simulink model "et_robocon_princess_pi_zack"  (R2013b)
settings: Solver=FixedStepDiscrete  SolverMode=SingleTasking  StartTime=0.0  StopTime=inf  FixedStep=balancer_ts  RelTol=1e-3
undefined symbols (not defined in the file): a_d, a_r, balancerStates_Bus0, Batt, battery_gain, battery_offset, cmd_max, current_mode_status, current_task_operation_status, DiscIntNeverNeededParam, exec_period, Init_Bus0, K, k_f, k_i, k_phidot, k_thetadot, lightCalib, R, see_saw_princess, STATE, TRACK_MODE_LIST, ts2, W
libraries: legonxtlib x29, simulink x19, simulink_extras x4
(part 4 of 4)

== system et_robocon_princess_pi_zack/Main Controller/normal_operation_modes.line_tracking_before_seesaw/line_tracking_mode.Track.lineTracker/SwitchForFreeSteering/tmpController/Derivative ==
  In : Inport
  Constant2 : Constant  Value=Ts_  OutDataTypeStr=single  SampleTime=-1
  Difference : simulink/Discrete/Difference  ICPrevInput=0.0  InputProcessing=Inherited  OutMin=[]  OutMax=[]  OutDataTypeStr=single  OutputDataTypeScalingMode=single  OutDataType=sfix(16)  OutScaling=2^-10  RndMeth=Nearest  DoSatur=off
  Divide4 : Product  Inputs=*/  OutDataTypeStr=single  RndMeth=Nearest
  Out : Outport
  wires:
  Constant2/1 -> Divide4/2
  Divide4/1 -> Difference/1
  In/1 -> Divide4/1
  Difference/1 -> Out/1

== system et_robocon_princess_pi_zack/Main Controller/normal_operation_modes.line_tracking_before_seesaw/line_tracking_mode.Track.lineTracker/SwitchForFreeSteering/tmpController/Fillter ==
  In : Inport
  In1 : Inport  Port=2
  Add : Sum  RndMeth=Nearest
  Add2 : Sum  Inputs=+-  OutDataTypeStr=single  RndMeth=Nearest
  Constant : Constant  Value=single(1-(0.0001/(0.1*Ts_)))  OutDataTypeStr=single  SampleTime=-1
  Constant1 : Constant  Value=single(0.0001/(0.1*Ts_))  OutDataTypeStr=single  SampleTime=-1
  Constant2 : Constant  Value=(0.1*Ts_)  OutDataTypeStr=single  SampleTime=-1
  Constant3 : Constant  OutDataTypeStr=single  SampleTime=-1
  Constant4 : Constant  Value=0.00001  OutDataTypeStr=single  SampleTime=-1
  Constant6 : Constant  Value=(0.1*Ts_)  OutDataTypeStr=single  SampleTime=-1
  Divide : Product  Inputs=*/
  Divide1 : Product  Inputs=*/
  Manual Switch1 : ManualSwitch  CurrentSetting=0
  Manual Switch3 : ManualSwitch  CurrentSetting=0
  Product : Product  OutDataTypeStr=single  RndMeth=Nearest
  Product1 : Product  OutDataTypeStr=single  RndMeth=Nearest
  Product3 : Product  OutDataTypeStr=single  RndMeth=Nearest
  Unit Delay : UnitDelay  SampleTime=-1
  Unit Delay1 : UnitDelay  SampleTime=-1
  Out : Outport
  wires:
  In/1 -> Unit Delay1/1
  Unit Delay1/1 -> Product1/1
  Product1/1 -> Add/1
  Unit Delay/1 -> Product/2
  Add/1 -> Out/1, Unit Delay/1
  Product/1 -> Add/2
  Constant6/1 -> Divide/2
  Constant2/1 -> Divide1/2
  Divide1/1 -> Add2/2
  In1/1 -> Product3/1
  Product3/1 -> Divide1/1, Divide/1
  Constant4/1 -> Product3/2
  Constant3/1 -> Add2/1
  Manual Switch1/1 -> Product1/2
  Constant1/1 -> Manual Switch1/1
  Divide/1 -> Manual Switch1/2
  Manual Switch3/1 -> Product/1
  Constant/1 -> Manual Switch3/1
  Add2/1 -> Manual Switch3/2

== system et_robocon_princess_pi_zack/Main Controller/normal_operation_modes.line_tracking_before_seesaw/line_tracking_mode.Track.lineTracker/SwitchForFreeSteering/tmpController/I_over_guard ==
  In1 : Inport
  Compare To Constant1 : simulink/Logic and Bit Operations/Compare To Constant  relop===  const=1  OutDataTypeStr=uint8
  Constant2 : Constant  Value=0  OutDataTypeStr=uint8  SampleTime=-1
  Constant4 : Constant  Value=0  OutDataTypeStr=uint8  SampleTime=-1
  Memory1 : Memory  X0=1  InheritSampleTime=on
  Switch : Switch  Threshold=1
  Out1 : Outport
  wires:
  Memory1/1 -> Compare To Constant1/1
  Constant2/1 -> Memory1/1
  Constant4/1 -> Switch/1
  Compare To Constant1/1 -> Switch/2
  Switch/1 -> Out1/1
  In1/1 -> Switch/3

== system et_robocon_princess_pi_zack/Main Controller/normal_operation_modes.line_tracking_before_seesaw/line_tracking_mode.Track.lineTracker/SwitchForFreeSteering/tmpController/Integrator ==
  In : Inport
  Constant2 : Constant  Value=Ts_  OutDataTypeStr=single  SampleTime=-1
  Integrator : DiscreteTransferFcn  Denominator=[1 -1]  RndMeth=Nearest
  Product1 : Product  OutDataTypeStr=single  RndMeth=Nearest
  Out : Outport
  wires:
  Constant2/1 -> Product1/2
  Product1/1 -> Integrator/1
  In/1 -> Product1/1
  Integrator/1 -> Out/1

== system et_robocon_princess_pi_zack/Main Controller/normal_operation_modes.line_tracking_before_seesaw/line_tracking_mode.balanceControl/ForSimulation/Cal_PWM/Cal_vol_max ==
  battery : Inport
  Constant : Constant  Value=battery_offset  OutDataTypeStr=single  SampleTime=-1
      settings: AttributesFormatString=DataType = %<OutDataTypeStr>
  Gain3 : Gain  Gain=battery_gain  OutDataTypeStr=Inherit: Same as input  ParamDataTypeStr=Inherit: Same as input
  Sum2 : Sum  Inputs=|+-  OutDataTypeStr=Inherit: Same as first input
  vol_max : Outport
  wires:
  Constant/1 -> Sum2/2
  Sum2/1 -> vol_max/1  "base_pwm"
  Gain3/1 -> Sum2/1
  battery/1 -> Gain3/1

== system et_robocon_princess_pi_zack/Main Controller/normal_operation_modes.line_tracking_before_seesaw/line_tracking_mode.balanceControl/ForSimulation/Cal_Reference/DiscreteIntegrator ==
  in : Inport
  Gain : Gain  Gain=exec_period  OutDataTypeStr=Inherit: Same as input  ParamDataTypeStr=Inherit: Same as input
  Sum : Sum  Inputs=|++  OutDataTypeStr=Inherit: Same as first input
  Unit Delay : UnitDelay  SampleTime=-1  StateName=ud_theta_ref  StateMustResolveToSignalObject=on
      settings: AttributesFormatString=Signal name = ud_theta_ref
  out : Outport
  wires:
  Unit Delay/1 -> Sum/2, out/1
  Gain/1 -> Sum/1
  Sum/1 -> Unit Delay/1
  in/1 -> Gain/1

== system et_robocon_princess_pi_zack/Main Controller/normal_operation_modes.line_tracking_before_seesaw/line_tracking_mode.balanceControl/ForSimulation/Cal_Reference/LowPathFilter ==
  note: Low Path Filter Function
      |               1-a_r
      |          ----------------
      |          1-a_r*z^(-1)
  in : Inport
  Constant : Constant  OutDataTypeStr=single
      settings: AttributesFormatString=DataType = %<OutDataTypeStr>
  Constant1 : Constant  Value=a_r  OutDataTypeStr=single
      settings: AttributesFormatString=DataType = %<OutDataTypeStr>
  Gain2 : Gain  Gain=a_r  OutDataTypeStr=Inherit: Same as input  ParamDataTypeStr=Inherit: Same as input
  Product : Product  RndMeth=Zero
  Sum : Sum  Inputs=|++  OutDataTypeStr=Inherit: Same as first input
  Sum1 : Sum  Inputs=|+-
  Unit Delay : UnitDelay  SampleTime=-1  StateName=ud_thetadot_cmd_lpf  StateMustResolveToSignalObject=on
      settings: AttributesFormatString=Signal name = ud_thetadot_cmd_lpf
  out : Outport
  wires:
  Sum/1 -> Unit Delay/1, out/1
  Unit Delay/1 -> Gain2/1
  Gain2/1 -> Sum/2
  Product/1 -> Sum/1
  in/1 -> Product/1
  Constant/1 -> Sum1/1
  Sum1/1 -> Product/2
  Constant1/1 -> Sum1/2

== system et_robocon_princess_pi_zack/Main Controller/normal_operation_modes.line_tracking_before_seesaw/line_tracking_mode.balanceControl/ForSimulation/Cal_x1/DiscreteDerivative ==
  in : Inport
  in1 : Inport  Port=2
  Constant : Constant  Value=exec_period  OutDataTypeStr=single
  Product : Product  Inputs=*/  RndMeth=Simplest
  Sum : Sum  Inputs=|+-  OutDataTypeStr=Inherit: Same as first input
  out : Outport
  wires:
  Sum/1 -> Product/1
  in1/1 -> Sum/2
  in/1 -> Sum/1
  Product/1 -> out/1
  Constant/1 -> Product/2

== system et_robocon_princess_pi_zack/Main Controller/normal_operation_modes.line_tracking_before_seesaw/line_tracking_mode.balanceControl/ForSimulation/Cal_x1/DiscreteIntegrator ==
  in : Inport
  Gain : Gain  Gain=exec_period  OutDataTypeStr=Inherit: Same as input  ParamDataTypeStr=Inherit: Same as input
  Sum : Sum  Inputs=|++  OutDataTypeStr=Inherit: Same as first input
  Unit Delay : UnitDelay  SampleTime=-1
      settings: AttributesFormatString=Signal name = ud_psi
  out : Outport
  wires:
  Unit Delay/1 -> Sum/2, out/1
  Gain/1 -> Sum/1
  Sum/1 -> Unit Delay/1
  in/1 -> Gain/1

== system et_robocon_princess_pi_zack/Main Controller/normal_operation_modes.line_tracking_before_seesaw/line_tracking_mode.balanceControl/ForSimulation/Cal_x1/LowPathFilter ==
  note: Low Path Filter Function
      |               1-a_d
      |          ----------------
      |          1-a_d*z^(-1)
  in : Inport
  Constant : Constant  OutDataTypeStr=single
      settings: AttributesFormatString=DataType = %<OutDataTypeStr>
  Constant1 : Constant  Value=a_d  OutDataTypeStr=single
      settings: AttributesFormatString=DataType = %<OutDataTypeStr>
  Gain2 : Gain  Gain=a_d  OutDataTypeStr=Inherit: Same as input  ParamDataTypeStr=Inherit: Same as input
  Product : Product  RndMeth=Zero
  Sum : Sum  Inputs=|++  OutDataTypeStr=Inherit: Same as first input
  Sum1 : Sum  Inputs=|+-
  Unit Delay : UnitDelay  SampleTime=-1  StateName=ud_theta_lpf  StateMustResolveToSignalObject=on
      settings: AttributesFormatString=Signal name = ud_thta_lpf
  out : Outport
  out1 : Outport  Port=2
  wires:
  Constant1/1 -> Sum1/2
  Sum1/1 -> Product/2
  Constant/1 -> Sum1/1
  in/1 -> Product/1
  Product/1 -> Sum/1
  Gain2/1 -> Sum/2
  Unit Delay/1 -> Gain2/1, out1/1
  Sum/1 -> out/1, Unit Delay/1  "theta_lpf"

== stateflow chart et_robocon_princess_pi_zack/State Estimation/Gyro Processing/Reset Subsystem ==
  state CheckForReset
    bind: doProcess;
    entry: doProcess;
    during: doProcess;
  (default) -> CheckForReset
  CheckForReset -> CheckForReset : [init_flag == 1]
  data: init_flag input
  events: doProcess output FUNCTION_CALL_EVENT

== stateflow chart et_robocon_princess_pi_zack/State Estimation/StateEstimation/Reset Subsystem ==
  state CheckForReset
    bind: doProcess;
    entry: doProcess;
    during: doProcess;
  (default) -> CheckForReset
  CheckForReset -> CheckForReset : [init_flag == 1]
  data: init_flag input
  events: doProcess output FUNCTION_CALL_EVENT

== stateflow chart et_robocon_princess_pi_zack/Main Controller/normal_operation_modes.see_saw_princess ==
  state see_saw_mode
    entry:
    desired_tail = single(1.6);
    during:
    normalizedLight = processLight(sensors.light,lightCalib);
    PWM.tail = tail_controller(sensors.theta_T, desired_tail);
    DispVar(normalizedLight);
    state light = processLight(rawLight,lightCalib) [function]
    state cmd = phiController(phi,desiredPhi,battery) [function]
    state Balancing
      state SeesawLogic [parallel]
        settings: executionOrder=1
        state StationnaryBalance
          entry:
          debugFlag = uint16(603);
          desired_tail = single(0.5);
          initFlags.theta = single(0);
          initFlags.gyroReset = single(0);
          desired_states = balancerStates_Bus0;
          phi0 = states.phi;
          desired_phi = phi0;
          during:
          %turningPWM = phiController(states.phi,desired_phi,sensors.battery);
          exit:
          turningPWM = single(0);
        state Seesaw
          entry:
          phi0 = states.phi;
          desired_phi = phi0;
          during:
          exit:
          turningPWM = single(0);
          note: % For now I store theta_ref when we receive the bluetooth signal.
              | Eventually one state needs to be added to sear for the ramp
              | and we should store the ref when the ramp is detected.
          state JumpOnIt
            entry:
            debugFlag = uint16(606);
            theta_ref = states.balancerStates.theta;
            des_vel = single(0.16);
            du:
            turningPWM = phiController(states.phi,desired_phi, sensors.battery);
          state ForPhi
            state GoingUP
              en:
              debugFlag = uint16(607);
              des_vel = single(0.1);
              du:
              turningPWM = phiController(states.phi,desired_phi, sensors.battery)+...
              single(3)*lineTracker(single(0.15), normalizedLight, single(1), sensors.battery);
              ex:
              des_vel = single(0);
            state WaitForMario
              en:
              debugFlag = uint16(608);
              des_vel = single(0);
              BT_status_out = single(102);
              du:
              turningPWM =phiController(states.phi,desired_phi, sensors.battery)
            state MoveForward
              en:
              debugFlag = uint16(609);
              des_vel = single(0.005);
              du:
              turningPWM = phiController(states.phi,desired_phi, sensors.battery)+...
              single(3)*lineTracker(single(0.3), normalizedLight, single(1), sensors.battery);
              ex:
              %des_vel = single(0.01);
              state Vel1
                du: des_vel = des_vel + single(0.00024);
              state Vel
                entry:
                des_vel = single(0.06)
                BT_status_out = single(103);
              (default) -> Vel1
              Vel1 -> Vel : [des_vel >= single(0.06)]
            state WaitForMario2
              en:
              debugFlag = uint16(610);
              BT_status_out = single(103);
              du:
              turningPWM =phiController(states.phi,desired_phi, sensors.battery);
            GoingUP -> WaitForMario : [states.balancerStates.theta >= theta_ref + single(5)]
            WaitForMario -> MoveForward : [sensors.BT_status_in == single(3)]
          state GetOff
            entry:
            debugFlag = uint16(611);
            des_vel = single(0);
            during:
            %turningPWM = single(1.1)*lineTracker(single(0.3), normalizedLight, single(1), sensors.battery)+single(1)*phiController(states.phi,desired_phi,sensors.battery);
            turningPWM = phiController(states.phi,desired_phi, sensors.battery);
            exit: des_vel = single(0.04);
          state Stop
            entry:
            debugFlag = uint16(612);
            BT_status_out = single(104);
            du:
            turningPWM = lineTracker(single(0), normalizedLight, single(1), sensors.battery);
            des_vel = des_vel + single(0.0003)
          state Stop1
            entry:
            debugFlag = uint16(613);
            du: turningPWM = lineTracker(single(0), normalizedLight, single(1), sensors.battery)
          (default) -> JumpOnIt
          JumpOnIt -> GoingUP : [states.balancerStates.theta >= theta_ref+single(1.8)]
          MoveForward -> GetOff : [sensors.BT_status_in == single(4)]
          GetOff -> GetOff : [states.balancerStates.theta >= theta_ref + single(30)]
          Stop -> Stop1 : [des_vel >= single(0.08)]
        state RaceDone
          entry: debugFlag = uint16(599);
          current_mode_status = OperationModeStatusEnum.SUCCESSFULLY_COMPLETED;
        (default) -> StationnaryBalance
        StationnaryBalance -> Seesaw
      state After [parallel]
        during:
        forwardPWM = balance_ctrl(states.balancerStates, des_vel ,sensors.battery)
        PWM.left = forwardPWM + turningPWM;
        PWM.right = forwardPWM - turningPWM;
        settings: executionOrder=2
    state cmd = lineTracker(desiredLight,light,trackingPower,battery) [function]
    state Speak [function]
    state cmd = tail_controller(current,desired) [function]
    state cmd = balance_ctrl(balancerStates,desired_velocity,battery) [function]
    state DispVar(Var) [function]
    (default) -> Balancing
  data: rawLight function_input single size=1; lightCalib function_input Bus: Light_Bus size=1; light function_output; cmd function_output; phi function_input single size=1; desiredPhi function_input single size=1; battery function_input double size=1; cmd function_output single size=1; desiredLight function_input single size=1; light function_input single size=1; trackingPower function_input single size=1; battery function_input double size=1; current function_input single size=1; desired function_input single size=1; cmd function_output single size=1; balancerStates function_input Bus: Balancer_States_Bus size=1; desired_velocity function_input single size=1; battery function_input double size=1; cmd function_output single size=1; Var function_input single size=1; states input Bus: States_Bus size=1; sensors input Bus: Sensors_Bus size=1; PWM output Bus: PWM_bus size=1; initFlags output Bus: Init_Bus size=1; debugFlag output uint16 size=1; desired_states local Bus: Balancer_States_Bus size=1; desired_tail local single size=1; current_mode_status data_store_memory; balancerStates_Bus0 parameter Bus: Balancer_States_Bus size=1; lightCalib data_store_memory; normalizedLight local single size=1; des_vel local single size=1; theta_ref local single size=1; forwardPWM local single size=1; turningPWM local single size=1; BT_status_out output single size=1; phi0 local single size=1; desired_phi local single size=1

== stateflow chart et_robocon_princess_pi_zack/Main Controller ==
  state restore
  state emergency_stop
    entry:
    debugFlag = uint16(9999);
  state normal_operation_modes
    state gyro_calibration_mode
    state light_calibration_up
    state line_tracking_before_seesaw
    state see_saw_princess
    state line_tracking_after_seesaw
    state WeShouldNotBeHere
    (default) -> (junction 12) : {
        | current_mode_status = OperationModeStatusEnum.IN_PROGRESS;
        | }
    (junction 12) -> gyro_calibration_mode [order 1] : [  current_mode == OperationModeEnum.GYRO_CALIBRATION ]
    (junction 12) -> (junction 13) [order 2]
    (junction 13) -> ? [order 1] : [ current_mode == OperationModeEnum.LIGHT_CALIBRATION_ON_TAIL ]
    (junction 13) -> (junction 144) [order 1]
    (junction 144) -> light_calibration_up [order 1] : [ current_mode == OperationModeEnum.LIGHT_CALIBRATION_UP ]
    (junction 144) -> (junction 14) [order 2]
    (junction 14) -> line_tracking_before_seesaw [order 2] : [ current_mode == OperationModeEnum.LINE_TRACKING ]
    (junction 14) -> (junction 15) [order 1]
    (junction 15) -> see_saw_princess [order 1] : [ current_mode == OperationModeEnum.SEE_SAW_PRINCESS ]
    (junction 15) -> (junction 17) [order 2]
    (junction 17) -> ? [order 1] : [  current_mode == OperationModeEnum.LIMBO ]
    (junction 17) -> (junction 19) [order 1]
    (junction 19) -> ? [order 1] : [ current_mode == OperationModeEnum.LIGHT_CALIBRATION_LIMBO ]
    (junction 19) -> (junction 140) [order 1]
    (junction 140) -> line_tracking_after_seesaw [order 1] : [ current_mode == OperationModeEnum.LINE_TRACKING_ON_MAP ]
    (junction 140) -> (junction 154) [order 2]
    (junction 154) -> ? [order 1] : [ current_mode == OperationModeEnum.YOSHI ]
    (junction 154) -> (junction 99) [order 1]
    (junction 99) -> WeShouldNotBeHere
  (default) -> (junction 38) : {initFlags = Init_Bus0;BT_status_out = single(0)}
  (junction 37) -> (junction 38)
  (junction 43) -> (junction 37)
  (junction 38) -> (junction 39) : { current_mode_index = uint8( 0 ); }
  (junction 40) -> (junction 39)
  restore -> (junction 40) : [ false == touch ]
  (junction 39) -> (junction 41) : {
      | current_mode_status = OperationModeStatusEnum.NOT_STARTED;
      | }
  normal_operation_modes -> (junction 40) [order 2] : [ current_mode_status == OperationModeStatusEnum.SUCCESSFULLY_COMPLETED ]
  (junction 42) -> (junction 41)
  (junction 41) -> (junction 44) : { current_mode_index = current_mode_index + uint8( 1 ); }
  (junction 47) -> (junction 42)
  emergency_stop -> restore : [ true == touch ]
  (junction 44) -> (junction 43) [order 1] : [ numel( TRACK_MODE_LIST ) < current_mode_index ]
      | % If the "current_mode_index" has exceeded the number
      | % of elements in the list, it should "wrap" back to the start.
  (junction 44) -> (junction 45) [order 2]
  (junction 45) -> (junction 46) : {
      | current_mode = TRACK_MODE_LIST( current_mode_index );
      | }
  (junction 46) -> (junction 47) [order 1] : [  current_mode == OperationModeEnum.SKIP ]
  (junction 46) -> normal_operation_modes [order 2]
  normal_operation_modes -> emergency_stop [order 1] : [ true == fall_detection_input ]
      | {current_mode_status = OperationModeStatusEnum.ABORTED;}
  data: rawSensors input Bus: Sensors_Bus size=1; PWM output Bus: PWM_bus size=1; TRACK_MODE_LIST parameter Enum: OperationModeEnum; current_mode_index local uint8; current_mode data_store_memory; states input Bus: States_Bus size=1; fall_detection_input input boolean size=1; current_mode_status data_store_memory; sensors input Bus: Sensors_Bus size=1; lightCalib data_store_memory; debugFlag output uint16 size=1; BT_status_out output single size=1; touch input single size=1; initFlags output Bus: Init_Bus size=1; Init_Bus0 parameter Bus: Init_Bus size=1; balancerStates_Bus0 parameter Bus: Balancer_States_Bus size=1

== stateflow chart et_robocon_princess_pi_zack/Main Controller/normal_operation_modes.line_tracking_after_seesaw ==
  state line_tracking_mode
    entry:
    desired_tail = single(0); %radian
    entry, during:
    PWM.tail = tail_controller(sensors.theta_T,desired_tail);
    exit:
    PWM.tail = single(0);
    state ResetStates
      entry:
      initFlags.theta = single(1);
      initFlags.gyroReset = single(1);
    state ResetDone
      entry:
      initFlags.theta = single(0);
      initFlags.gyroReset = single(0);
    state Track
      entry:
      debugFlag = uint16(401);
      bias = single(0);
      FlagSteering = single(0);
      minLight = single(-125);
      maxLight = single(-10);
      lineSide = single(1);
      enablePhiTracking = single(0);
      state preProcess [parallel]
        during:
        on every(3, tick):
        [normalizedLight, filteredLight] = processLight(sensors.light, bias, minLight,maxLight);
        [AngleCount,EncoderReset,Angle, Distance] = analyzeEncoders(rawSensors);
        settings: executionOrder=1
      state manageRacePhases [parallel]
        settings: executionOrder=2
        state ApproahSeesawtransition3
          entry:
          Speak;
          PID = single([0 0 0 0 0]');
          bias = single(0);
          FlagSteering = single(1);
          lineSide = single(-1);
          phi_tmp  =single(0);
          enablePhiTracking = single(1);
          state accelerate1
            during:
            fwd = fwd + single(1/3);
          state coast1
          (default) -> line_tracking_mode.Track.manageRacePhases.ApproahSeesawtransition3.accelerate1
          line_tracking_mode.Track.manageRacePhases.ApproahSeesawtransition3.accelerate1 -> line_tracking_mode.Track.manageRacePhases.ApproahSeesawtransition3.coast1 : [fwd >= 20]
        state SlowlyRestartLineTracking
          entry: Speak;
          PID = single([30 0 25 0 100]');
          bias = single(0);
          FlagSteering = single(0);
          enablePhiTracking = single(0);
        state Bypass
          entry:
          Speak;
          PID = single([30 0 25 0 100]');
          FlagSteering = single(0);
          enablePhiTracking = single(0);
          state accelerate
            during:
            fwd = fwd + single(1/3);
          state coast
          (default) -> accelerate
          accelerate -> coast : [fwd >= 80]
        state ApproahSeesawtransition2
          entry:
          Speak;
          PID = single([30 0 25 0 100]');
          FlagSteering = single(0);
          lineSide = single(-1);
          state accelerate1
            during:
            fwd = fwd - single(1/3);
          state coast1
          (default) -> line_tracking_mode.Track.manageRacePhases.ApproahSeesawtransition2.accelerate1
          line_tracking_mode.Track.manageRacePhases.ApproahSeesawtransition2.accelerate1 -> line_tracking_mode.Track.manageRacePhases.ApproahSeesawtransition2.coast1 : [fwd <= 0]
        (default) -> ApproahSeesawtransition3
        ApproahSeesawtransition3 -> SlowlyRestartLineTracking : [filteredLight>(maxLight + minLight)/2]
        SlowlyRestartLineTracking -> Bypass : after(1,sec)
        Bypass -> ApproahSeesawtransition2 : [Distance >= single(8*360)]
      state ApplyControl [parallel]
        during:
        on every(3, tick):  lineTrackCmd = lineTracker(normalizedLight,FlagSteering,PID,fwd)
        during:
        %lineTrackCmd(2) = lineSide*lineTrackCmd(2);
        if lineSide >0
        [PWM.left PWM.right] = balanceControl(rawSensors,lineTrackCmd);
        if enablePhiTracking
        PWM.left = PWM.left + phiController(states.phi,phi_tmp,sensors.battery);
        PWM.right = PWM.right - phiController(states.phi,phi_tmp,sensors.battery);
        end
        else
        [PWM.right PWM.left] = balanceControl(rawSensors,lineTrackCmd);
        if enablePhiTracking
        PWM.left = PWM.left + phiController(states.phi,phi_tmp,sensors.battery);
        PWM.right = PWM.right - phiController(states.phi,phi_tmp,sensors.battery);
        end
        end
        dispL5(states.balancerStates.theta_dot);
        settings: executionOrder=3
      state [normalizedLight,filteredLight] = processLight(rawLight,bias,minLight,maxLight) [function]
      state [AngleCount,EncoderReset,Angle,Distance] = analyzeEncoders(rawSensors) [function]
      state cmd = lineTracker(lightSignal,flagSteering,PID,fwd) [function]
      state dispL5(x) [function]
    state SitDown
      state Stop
        during:
        lineTrackCmd = single([0 0]');
        [PWM.left PWM.right] = balanceControl(rawSensors,lineTrackCmd);
        desired_tail = single(1.6); %radian
      state Kick
        entry:
        PWM.left = single(100)
        PWM.right = single(100);
        exit:
        PWM.left = single(0)
        PWM.right = single(0);
      state Done
        entry:
        turnLightOn;
        debugFlag = uint16(402);
        PWM.left = single(0); PWM.right = single(0);
        %current_mode_status = OperationModeStatusEnum.SUCCESSFULLY_COMPLETED;
      (default) -> Stop
      Stop -> Kick : after(0.5,sec)
      Kick -> Done : after(0.2,sec)
    state cmd = phiController(phi,desiredPhi,battery) [function]
    state [leftPWM,rightPWM]  = balanceControl(rawSensors, lineTrackCmd) [function]
    state cmd = tail_controller(current,desired) [function]
    state turnLightOn [function]
    state Speak [function]
    (default) -> ResetStates
    ResetStates -> ResetDone
    ResetDone -> Track
    ApproahSeesawtransition2 -> SitDown : after(2,sec)
  data: rawLight function_input single size=1; bias function_input single size=1; normalizedLight function_output single size=1; filteredLight function_output single size=1; minLight function_input single size=1; maxLight function_input single size=1; rawSensors function_input Bus: Sensors_Bus size=1; AngleCount function_output uint8 size=1; EncoderReset function_output single size=1; Angle function_output single size=1; Distance function_output single size=1; lightSignal function_input single size=1; flagSteering function_input single size=1; PID function_input single size=5; fwd function_input single size=1; cmd function_output; x function_input double size=1; cmd function_output; phi function_input single size=1; desiredPhi function_input single size=1; battery function_input double size=1; leftPWM function_output single size=1; rawSensors function_input Bus: Sensors_Bus size=1; rightPWM function_output; lineTrackCmd function_input single size=2; current function_input single size=1; desired function_input single size=1; cmd function_output single size=1; sensors input Bus: Sensors_Bus size=1; touch input single size=1; PWM output Bus: PWM_bus size=1; debugFlag output uint16 size=1; current_mode_status data_store_memory; desired_tail local single size=1; speed_ref local single size=1; states input Bus: States_Bus size=1; rawSensors input Bus: Sensors_Bus size=1; lineTrackCmd local single size=2; PID local single size=5; normalizedLight local single size=1; AngleCount local uint8 size=1; EncoderReset local single size=1; Angle local single size=1; bias local single size=1; fwd local single size=1; FlagSteering local single size=1; filteredLight local single; EncoderTmp local single size=1; Distance local single size=1; minLight local; maxLight local; phi_tmp local single size=1; enablePhiTracking local; d0 local; lineSide local; theta_ref local; initFlags output Bus: Init_Bus size=1

== stateflow chart et_robocon_princess_pi_zack/Main Controller/normal_operation_modes.light_calibration_up ==
  state wait
    entry:debugFlag = uint16(200);
  state MoveUp
    entry:debugFlag = uint16(201);
    PWM.tail = single(-50);
  state Reset
    entry:debugFlag = uint16(202);
    PWM.tail = single(0);
    initFlags.tail = single(1);
    exit:
    initFlags.tail = single(0);
    desired_tail = single(0);
  state light_sensor_calibration_up
    %during, exit: PWM.tail = tail_controller(sensors.theta_T,single(1.6))
    state WaitForBlack
      entry: debugFlag = uint16(310);
    state StoreBlack
      entry: lightCalib.black = sensors.light;
      debugFlag = uint16(311);
    state WaitForWhite
      entry: debugFlag = uint16(312)
    state StoreWhite
      entry: lightCalib.white = sensors.light;
      debugFlag = uint16(313);
    state CalibComplete
      entry:
      debugFlag = uint16(318);
      current_task_operation_status = OperationModeStatusEnum.SUCCESSFULLY_COMPLETED;
    state cmd = tail_controller(current,desired) [function]
    (default) -> WaitForBlack
    WaitForBlack -> StoreBlack : [hasChangedFrom(touch,single(0))]
    StoreBlack -> WaitForWhite : after(1,sec)
    WaitForWhite -> StoreWhite : [hasChangedFrom(touch,single(0))]
    StoreWhite -> CalibComplete : after(1,sec)
  (default) -> wait
  wait -> MoveUp : [hasChangedFrom(touch,single(0))]
  MoveUp -> Reset : after(2,sec)
  Reset -> light_sensor_calibration_up : after(1,sec)
  data: current function_input single size=1; desired function_input single size=1; cmd function_output single size=1; sensors input Bus: Sensors_Bus size=1; lightCalib data_store_memory; current_task_operation_status data_store_memory; debugFlag output uint16; touch input single size=1; PWM output Bus: PWM_bus size=1; initFlags output Bus: Init_Bus size=1; desired_tail local
